simulink model "db3_6_Level_double"  (R2021a)
settings: Solver=VariableStepAuto  StartTime=0.0  StopTime=8  RelTol=1e-3
undefined symbols (not defined in the file): lambda2
libraries: dspsigops x13, dspquant2 x1
(part 1 of 3)
settings Model: Creator=Ruth Matienzo  LastModifiedBy=Ruth Matienzo

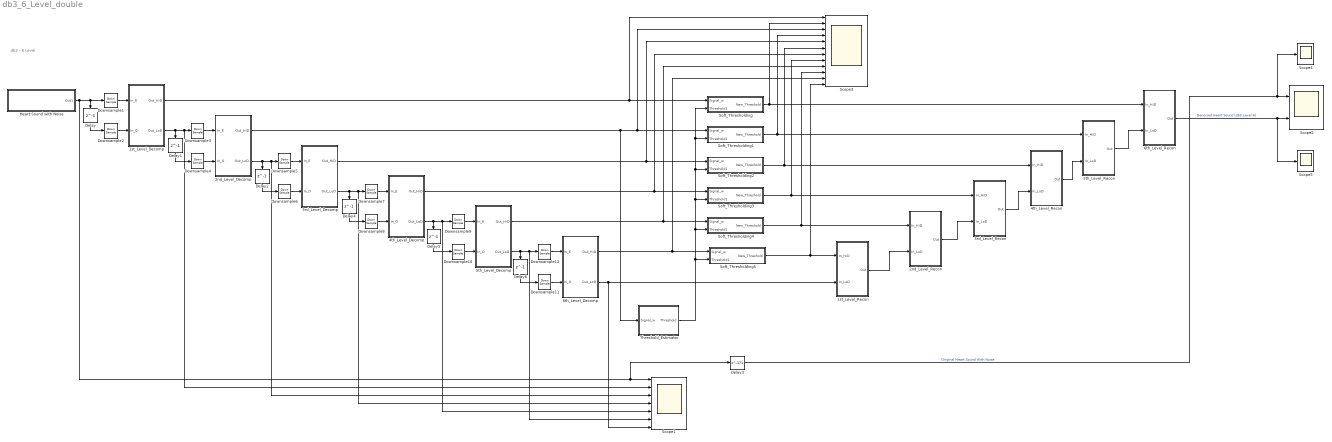
== system db3_6_Level_double ==
  note: db3 - 6 Level
  1st_Level_Decomp : Subsystem
  1st_Level_Recon : Subsystem
  2nd_Level_Decomp : Subsystem
  2nd_Level_Recon : Subsystem
  3rd_Level_Decomp : Subsystem
  3rd_Level_Recon : Subsystem
  4th_Level_Decomp : Subsystem
  4th_Level_Recon : Subsystem
  5th_Level_Decomp : Subsystem
  5th_Level_Recon : Subsystem
  6th_Level_Decomp : Subsystem
  6th_Level_Recon : Subsystem
  Delay{,1..2,4..6} (6 alike) : Delay  DelayLength=1  SampleTime=1/44100
  Delay3 : Delay  DelayLength=171  SampleTime=1/44100
  Downsample{1..12} (12 alike) : DownSample  N=30
  Heart Sound with Noise : Subsystem
  Scope1 : Scope  NumInputPorts=7
  Scope2 : Scope  NumInputPorts=2
  Scope3 : Scope  NumInputPorts=12
  Scope4 : Scope
  Scope5 : Scope
  Soft_Thresholding : Subsystem
  Soft_Thresholding1 : Subsystem
  Soft_Thresholding2 : Subsystem
  Soft_Thresholding3 : Subsystem
  Soft_Thresholding4 : Subsystem
  Soft_Thresholding5 : Subsystem
  Threshold_Estimator : Subsystem
  wires:
  1st_Level_Decomp/2(Out_LoD) -> Scope1/2, Downsample3/1, Delay1/1
  Downsample5/1 -> 3rd_Level_Decomp/1(In_E)
  Downsample8/1 -> 4th_Level_Decomp/2(In_O)
  Heart Sound with Noise/1(Out1) -> Downsample1/1, Delay/1, Delay3/1, Scope1/1
  Downsample3/1 -> 2nd_Level_Decomp/1(In_E)
  Delay2/1 -> Downsample6/1
  Downsample1/1 -> 1st_Level_Decomp/1(In_E)
  2nd_Level_Decomp/1(Out_HiD) -> Threshold_Estimator/1(Signal_w), Soft_Thresholding1/1(Signal_w), Scope3/3
  1st_Level_Decomp/1(Out_HiD) -> Soft_Thresholding/1(Signal_w), Scope3/1
  Soft_Thresholding1/1(New_Threshold) -> 5th_Level_Recon/1(In_HiD), Scope3/4
  Soft_Thresholding2/1(New_Threshold) -> 4th_Level_Recon/1(In_HiD), Scope3/6
  Downsample7/1 -> 4th_Level_Decomp/1(In_E)
  Soft_Thresholding/1(New_Threshold) -> 6th_Level_Recon/1(In_HiD), Scope3/2
  Downsample2/1 -> 1st_Level_Decomp/2(In_O)
  Downsample6/1 -> 3rd_Level_Decomp/2(In_O)
  Delay4/1 -> Downsample8/1
  Soft_Thresholding3/1(New_Threshold) -> 3rd_Level_Recon/1(In_HiD), Scope3/8
  Delay/1 -> Downsample2/1
  3rd_Level_Decomp/1(Out_HiD) -> Soft_Thresholding2/1(Signal_w), Scope3/5
  3rd_Level_Recon/1(Out) -> 4th_Level_Recon/2(In_LoD)
  4th_Level_Decomp/1(Out_HiD) -> Soft_Thresholding3/1(Signal_w), Scope3/7
  5th_Level_Recon/1(Out) -> 6th_Level_Recon/2(In_LoD)
  Downsample9/1 -> 5th_Level_Decomp/1(In_E)
  Delay5/1 -> Downsample10/1
  2nd_Level_Decomp/2(Out_LoD) -> Scope1/3, Downsample5/1, Delay2/1
  4th_Level_Recon/1(Out) -> 5th_Level_Recon/2(In_LoD)
  Threshold_Estimator/1(Threshold) -> Soft_Thresholding4/2(Threshold1), Soft_Thresholding1/2(Threshold1), Soft_Thresholding/2(Threshold1), Soft_Thresholding2/2(Threshold1), Soft_Thresholding3/2(Threshold1), Soft_Thresholding5/2(Threshold1)
  Delay1/1 -> Downsample4/1
  3rd_Level_Decomp/2(Out_LoD) -> Scope1/4, Downsample7/1, Delay4/1
  Downsample4/1 -> 2nd_Level_Decomp/2(In_O)
  Downsample10/1 -> 5th_Level_Decomp/2(In_O)
  4th_Level_Decomp/2(Out_LoD) -> Scope1/5, Downsample9/1, Delay5/1
  2nd_Level_Recon/1(Out) -> 3rd_Level_Recon/2(In_LoD)
  Soft_Thresholding4/1(New_Threshold) -> 2nd_Level_Recon/1(In_HiD), Scope3/10
  5th_Level_Decomp/1(Out_HiD) -> Scope3/9, Soft_Thresholding4/1(Signal_w)
  5th_Level_Decomp/2(Out_LoD) -> Scope1/6, Downsample12/1, Delay6/1
  Downsample11/1 -> 6th_Level_Decomp/2(In_O)
  Delay6/1 -> Downsample11/1
  Downsample12/1 -> 6th_Level_Decomp/1(In_E)
  6th_Level_Decomp/2(Out_LoD) -> 1st_Level_Recon/2(In_LoD), Scope1/7
  6th_Level_Decomp/1(Out_HiD) -> Scope3/11, Soft_Thresholding5/1(Signal_w)
  Soft_Thresholding5/1(New_Threshold) -> 1st_Level_Recon/1(In_HiD), Scope3/12
  1st_Level_Recon/1(Out) -> 2nd_Level_Recon/2(In_LoD)
  Delay3/1 -> Scope4/1, Scope2/1  "Original Heart Sound With Noise"
  6th_Level_Recon/1(Out) -> Scope5/1, Scope2/2  "Denoised Heart Sound (db3 Level 6)"

== system db3_6_Level_double/1st_Level_Decomp ==
  In_E : Inport  OutDataTypeStr=double  SampleTime=1/44100
  In_O : Inport  Port=2  OutDataTypeStr=double  SampleTime=1/44100
  Add : Sum  AccumDataTypeStr=double  OutDataTypeStr=double
  Add1 : Sum  AccumDataTypeStr=double  OutDataTypeStr=double
  Delay1 : Delay  DelayLength=1  SampleTime=1/44100
  Delay2 : Delay  DelayLength=1  SampleTime=1/44100
  Divide1 : Product  Inputs=*/  OutDataTypeStr=double
  Divide2 : Product  Inputs=*/  OutDataTypeStr=double
  HiD : Constant  Value=0.877989329+0.977128821  OutDataTypeStr=double  SampleTime=1/44100
  HiD_Even : Subsystem
  HiD_Odd : Subsystem
  LoD : Constant  Value=0.977128821+0.877989329  OutDataTypeStr=double  SampleTime=1/44100
  LoD_Even : Subsystem
  LoD_Odd : Subsystem
  Out_HiD : Outport  OutDataTypeStr=double  SampleTime=1/44100
  Out_LoD : Outport  Port=2  OutDataTypeStr=double  SampleTime=1/44100
  wires:
  HiD_Even/1(Out_HiD_e) -> Add/1
  HiD_Odd/1(Out_HiD_o) -> Add/2
  LoD_Odd/1(Out_LoD_o) -> Add1/2
  LoD_Even/1(Out_LoD_e) -> Add1/1
  In_E/1 -> HiD_Even/1(In_HiD_e), LoD_Even/1(In_LoD_e)
  In_O/1 -> LoD_Odd/1(In_LoD_o), HiD_Odd/1(In_HiD_o)
  HiD/1 -> Divide1/2
  Add1/1 -> Divide2/1
  LoD/1 -> Divide2/2
  Add/1 -> Divide1/1
  Delay1/1 -> Out_HiD/1
  Divide1/1 -> Delay1/1
  Delay2/1 -> Out_LoD/1
  Divide2/1 -> Delay2/1

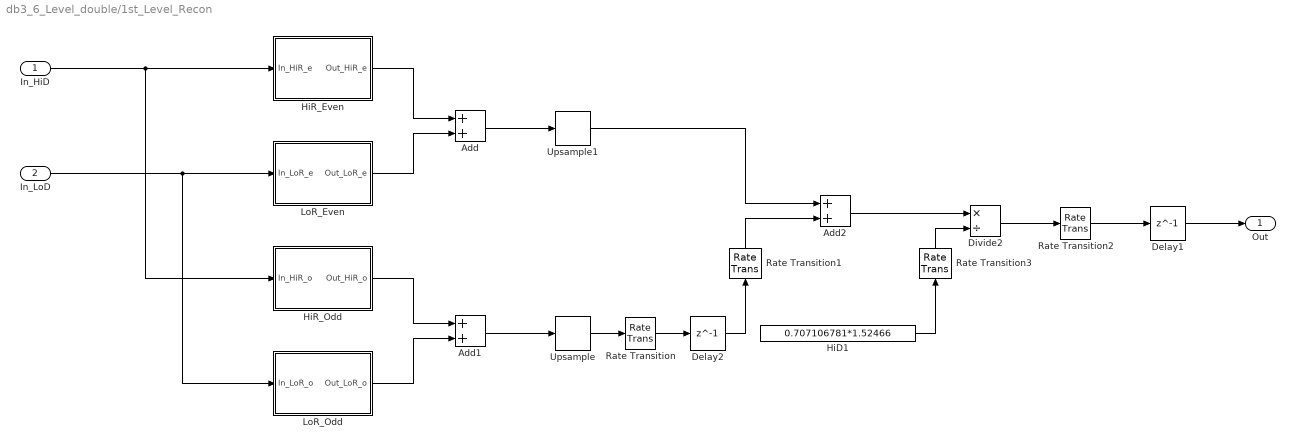
== system db3_6_Level_double/1st_Level_Recon ==
  In_HiD : Inport  OutDataTypeStr=double  SampleTime=1/44100
  In_LoD : Inport  Port=2  OutDataTypeStr=double  SampleTime=1/44100
  Add : Sum  AccumDataTypeStr=double  OutDataTypeStr=double
  Add1 : Sum  AccumDataTypeStr=double  OutDataTypeStr=double
  Add2 : Sum  AccumDataTypeStr=double  OutDataTypeStr=double
  Delay1 : Delay  DelayLength=1  SampleTime=1/44100
  Delay2 : Delay  DelayLength=1  SampleTime=1/44100
  Divide2 : Product  Inputs=*/  OutDataTypeStr=double  RndMeth=Zero  SaturateOnIntegerOverflow=on
  HiD1 : Constant  Value=0.707106781*1.52466  OutDataTypeStr=double  SampleTime=1/44100
  HiR_Even : Subsystem
  HiR_Odd : Subsystem
  LoR_Even : Subsystem
  LoR_Odd : Subsystem
  Rate Transition{,1..3} (4 alike) : RateTransition  OutPortSampleTime=1/44100
  Upsample : dspsigops/Upsample  N=30  phase=0  RateOptions=Allow multirate processing  ic=0  mode=Unused parameter value
  Upsample1 : dspsigops/Upsample  N=30  phase=0  RateOptions=Allow multirate processing  ic=0  mode=Unused parameter value
  Out : Outport  OutDataTypeStr=double  SampleTime=1/44100
  wires:
  In_HiD/1 -> HiR_Odd/1(In_HiR_o), HiR_Even/1(In_HiR_e)
  Add/1 -> Upsample1/1
  Add1/1 -> Upsample/1
  Upsample/1 -> Rate Transition/1
  Upsample1/1 -> Add2/1
  Delay2/1 -> Rate Transition1/1
  HiR_Even/1(Out_HiR_e) -> Add/1
  In_LoD/1 -> LoR_Odd/1(In_LoR_o), LoR_Even/1(In_LoR_e)
  LoR_Even/1(Out_LoR_e) -> Add/2
  HiR_Odd/1(Out_HiR_o) -> Add1/1
  LoR_Odd/1(Out_LoR_o) -> Add1/2
  Rate Transition/1 -> Delay2/1
  Rate Transition1/1 -> Add2/2
  Rate Transition2/1 -> Delay1/1
  Delay1/1 -> Out/1
  HiD1/1 -> Rate Transition3/1
  Add2/1 -> Divide2/1
  Divide2/1 -> Rate Transition2/1
  Rate Transition3/1 -> Divide2/2

== system db3_6_Level_double/2nd_Level_Decomp ==
  In_E : Inport  OutDataTypeStr=double  SampleTime=1/44100
  In_O : Inport  Port=2  OutDataTypeStr=double  SampleTime=1/44100
  Add : Sum  AccumDataTypeStr=double  OutDataTypeStr=double
  Add1 : Sum  AccumDataTypeStr=double  OutDataTypeStr=double
  Delay1 : Delay  DelayLength=1  SampleTime=1/44100
  Delay2 : Delay  DelayLength=1  SampleTime=1/44100
  Divide1 : Product  Inputs=*/  OutDataTypeStr=double
  Divide2 : Product  Inputs=*/  OutDataTypeStr=double
  HiD : Constant  Value=0.877989329+0.977128821  OutDataTypeStr=double  SampleTime=1/44100
  HiD_Even : Subsystem
  HiD_Odd : Subsystem
  LoD : Constant  Value=0.977128821+0.877989329  OutDataTypeStr=double  SampleTime=1/44100
  LoD_Even : Subsystem
  LoD_Odd : Subsystem
  Out_HiD : Outport  OutDataTypeStr=double  SampleTime=1/44100
  Out_LoD : Outport  Port=2  OutDataTypeStr=double  SampleTime=1/44100
  wires:
  HiD_Even/1(Out_HiD_e) -> Add/1
  HiD_Odd/1(Out_HiD_o) -> Add/2
  LoD_Odd/1(Out_LoD_o) -> Add1/2
  LoD_Even/1(Out_LoD_e) -> Add1/1
  In_E/1 -> HiD_Even/1(In_HiD_e), LoD_Even/1(In_LoD_e)
  In_O/1 -> LoD_Odd/1(In_LoD_o), HiD_Odd/1(In_HiD_o)
  HiD/1 -> Divide1/2
  Add1/1 -> Divide2/1
  LoD/1 -> Divide2/2
  Add/1 -> Divide1/1
  Delay1/1 -> Out_HiD/1
  Divide1/1 -> Delay1/1
  Delay2/1 -> Out_LoD/1
  Divide2/1 -> Delay2/1

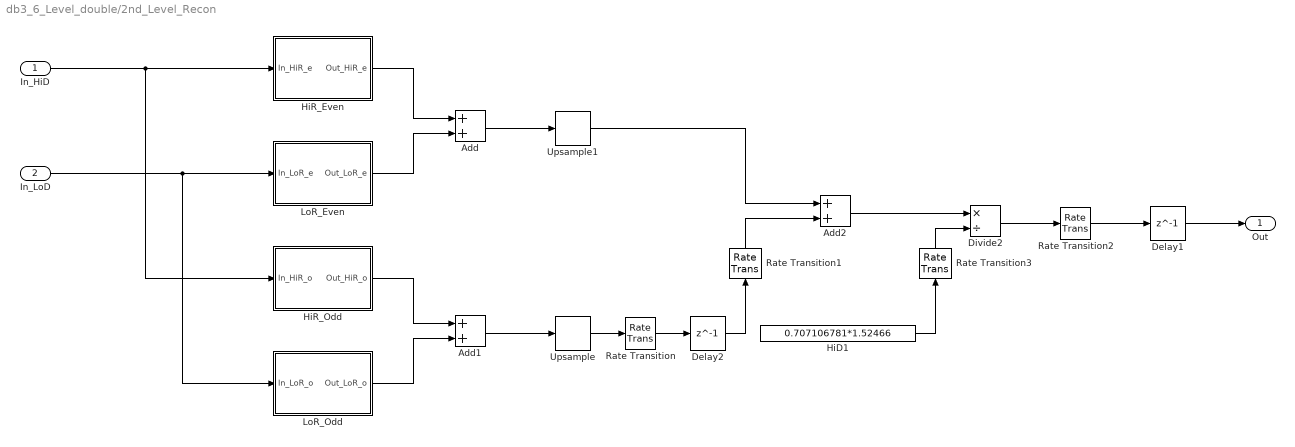
== system db3_6_Level_double/2nd_Level_Recon ==
  In_HiD : Inport  OutDataTypeStr=double  SampleTime=1/44100
  In_LoD : Inport  Port=2  OutDataTypeStr=double  SampleTime=1/44100
  Add : Sum  AccumDataTypeStr=double  OutDataTypeStr=double
  Add1 : Sum  AccumDataTypeStr=double  OutDataTypeStr=double
  Add2 : Sum  AccumDataTypeStr=double  OutDataTypeStr=double
  Delay1 : Delay  DelayLength=1  SampleTime=1/44100
  Delay2 : Delay  DelayLength=1  SampleTime=1/44100
  Divide2 : Product  Inputs=*/  OutDataTypeStr=double  RndMeth=Zero  SaturateOnIntegerOverflow=on
  HiD1 : Constant  Value=0.707106781*1.52466  OutDataTypeStr=double  SampleTime=1/44100
  HiR_Even : Subsystem
  HiR_Odd : Subsystem
  LoR_Even : Subsystem
  LoR_Odd : Subsystem
  Rate Transition{,1..3} (4 alike) : RateTransition  OutPortSampleTime=1/44100
  Upsample : dspsigops/Upsample  N=30  phase=0  RateOptions=Allow multirate processing  ic=0  mode=Unused parameter value
  Upsample1 : dspsigops/Upsample  N=30  phase=0  RateOptions=Allow multirate processing  ic=0  mode=Unused parameter value
  Out : Outport  OutDataTypeStr=double  SampleTime=1/44100
  wires:
  In_HiD/1 -> HiR_Odd/1(In_HiR_o), HiR_Even/1(In_HiR_e)
  Add/1 -> Upsample1/1
  Add1/1 -> Upsample/1
  Upsample/1 -> Rate Transition/1
  Upsample1/1 -> Add2/1
  Delay2/1 -> Rate Transition1/1
  HiR_Even/1(Out_HiR_e) -> Add/1
  In_LoD/1 -> LoR_Odd/1(In_LoR_o), LoR_Even/1(In_LoR_e)
  LoR_Even/1(Out_LoR_e) -> Add/2
  HiR_Odd/1(Out_HiR_o) -> Add1/1
  LoR_Odd/1(Out_LoR_o) -> Add1/2
  Rate Transition/1 -> Delay2/1
  Rate Transition1/1 -> Add2/2
  Rate Transition2/1 -> Delay1/1
  Delay1/1 -> Out/1
  HiD1/1 -> Rate Transition3/1
  Add2/1 -> Divide2/1
  Divide2/1 -> Rate Transition2/1
  Rate Transition3/1 -> Divide2/2

== system db3_6_Level_double/3rd_Level_Decomp ==
  In_E : Inport  OutDataTypeStr=double  SampleTime=1/44100
  In_O : Inport  Port=2  OutDataTypeStr=double  SampleTime=1/44100
  Add : Sum  AccumDataTypeStr=double  OutDataTypeStr=double
  Add1 : Sum  AccumDataTypeStr=double  OutDataTypeStr=double
  Delay1 : Delay  DelayLength=1  SampleTime=1/44100
  Delay2 : Delay  DelayLength=1  SampleTime=1/44100
  Divide1 : Product  Inputs=*/  OutDataTypeStr=double
  Divide2 : Product  Inputs=*/  OutDataTypeStr=double
  HiD : Constant  Value=0.877989329+0.977128821  OutDataTypeStr=double  SampleTime=1/44100
  HiD_Even : Subsystem
  HiD_Odd : Subsystem
  LoD : Constant  Value=0.977128821+0.877989329  OutDataTypeStr=double  SampleTime=1/44100
  LoD_Even : Subsystem
  LoD_Odd : Subsystem
  Out_HiD : Outport  OutDataTypeStr=double  SampleTime=1/44100
  Out_LoD : Outport  Port=2  OutDataTypeStr=double  SampleTime=1/44100
  wires:
  HiD_Even/1(Out_HiD_e) -> Add/1
  HiD_Odd/1(Out_HiD_o) -> Add/2
  LoD_Odd/1(Out_LoD_o) -> Add1/2
  LoD_Even/1(Out_LoD_e) -> Add1/1
  In_E/1 -> HiD_Even/1(In_HiD_e), LoD_Even/1(In_LoD_e)
  In_O/1 -> LoD_Odd/1(In_LoD_o), HiD_Odd/1(In_HiD_o)
  HiD/1 -> Divide1/2
  Add1/1 -> Divide2/1
  LoD/1 -> Divide2/2
  Add/1 -> Divide1/1
  Delay1/1 -> Out_HiD/1
  Divide1/1 -> Delay1/1
  Delay2/1 -> Out_LoD/1
  Divide2/1 -> Delay2/1

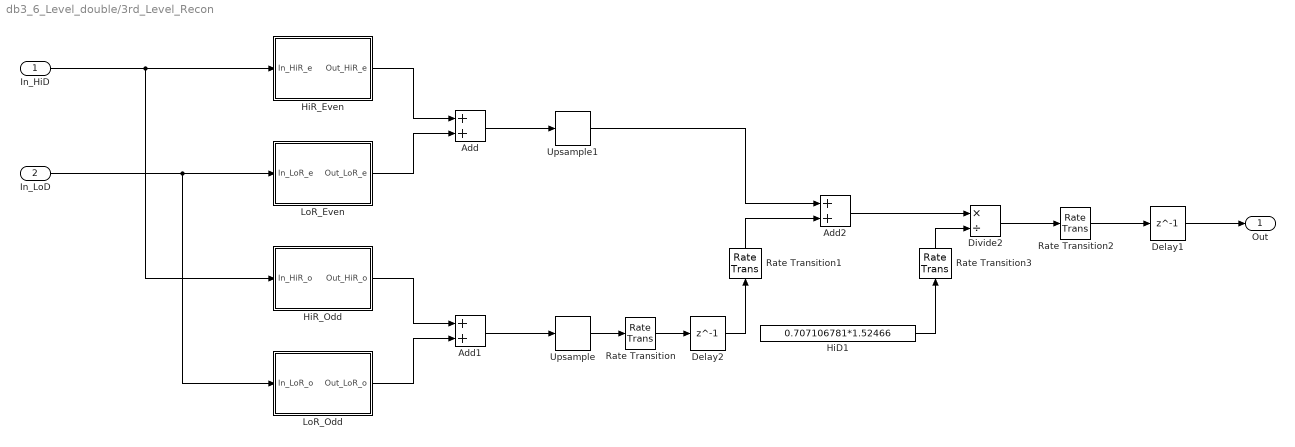
== system db3_6_Level_double/3rd_Level_Recon ==
  In_HiD : Inport  OutDataTypeStr=double  SampleTime=1/44100
  In_LoD : Inport  Port=2  OutDataTypeStr=double  SampleTime=1/44100
  Add : Sum  AccumDataTypeStr=double  OutDataTypeStr=double
  Add1 : Sum  AccumDataTypeStr=double  OutDataTypeStr=double
  Add2 : Sum  AccumDataTypeStr=double  OutDataTypeStr=double
  Delay1 : Delay  DelayLength=1  SampleTime=1/44100
  Delay2 : Delay  DelayLength=1  SampleTime=1/44100
  Divide2 : Product  Inputs=*/  OutDataTypeStr=double  RndMeth=Zero  SaturateOnIntegerOverflow=on
  HiD1 : Constant  Value=0.707106781*1.52466  OutDataTypeStr=double  SampleTime=1/44100
  HiR_Even : Subsystem
  HiR_Odd : Subsystem
  LoR_Even : Subsystem
  LoR_Odd : Subsystem
  Rate Transition{,1..3} (4 alike) : RateTransition  OutPortSampleTime=1/44100
  Upsample : dspsigops/Upsample  N=30  phase=0  RateOptions=Allow multirate processing  ic=0  mode=Unused parameter value
  Upsample1 : dspsigops/Upsample  N=30  phase=0  RateOptions=Allow multirate processing  ic=0  mode=Unused parameter value
  Out : Outport  OutDataTypeStr=double  SampleTime=1/44100
  wires:
  In_HiD/1 -> HiR_Odd/1(In_HiR_o), HiR_Even/1(In_HiR_e)
  Add/1 -> Upsample1/1
  Add1/1 -> Upsample/1
  Upsample/1 -> Rate Transition/1
  Upsample1/1 -> Add2/1
  Delay2/1 -> Rate Transition1/1
  HiR_Even/1(Out_HiR_e) -> Add/1
  In_LoD/1 -> LoR_Odd/1(In_LoR_o), LoR_Even/1(In_LoR_e)
  LoR_Even/1(Out_LoR_e) -> Add/2
  HiR_Odd/1(Out_HiR_o) -> Add1/1
  LoR_Odd/1(Out_LoR_o) -> Add1/2
  Rate Transition/1 -> Delay2/1
  Rate Transition1/1 -> Add2/2
  Rate Transition2/1 -> Delay1/1
  Delay1/1 -> Out/1
  HiD1/1 -> Rate Transition3/1
  Add2/1 -> Divide2/1
  Divide2/1 -> Rate Transition2/1
  Rate Transition3/1 -> Divide2/2

== system db3_6_Level_double/4th_Level_Decomp ==
  In_E : Inport  OutDataTypeStr=double  SampleTime=1/44100
  In_O : Inport  Port=2  OutDataTypeStr=double  SampleTime=1/44100
  Add : Sum  AccumDataTypeStr=double  OutDataTypeStr=double
  Add1 : Sum  AccumDataTypeStr=double  OutDataTypeStr=double
  Delay1 : Delay  DelayLength=1  SampleTime=1/44100
  Delay2 : Delay  DelayLength=1  SampleTime=1/44100
  Divide1 : Product  Inputs=*/  OutDataTypeStr=double
  Divide2 : Product  Inputs=*/  OutDataTypeStr=double
  HiD : Constant  Value=0.877989329+0.977128821  OutDataTypeStr=double  SampleTime=1/44100
  HiD_Even : Subsystem
  HiD_Odd : Subsystem
  LoD : Constant  Value=0.977128821+0.877989329  OutDataTypeStr=double  SampleTime=1/44100
  LoD_Even : Subsystem
  LoD_Odd : Subsystem
  Out_HiD : Outport  OutDataTypeStr=double  SampleTime=1/44100
  Out_LoD : Outport  Port=2  OutDataTypeStr=double  SampleTime=1/44100
  wires:
  HiD_Even/1(Out_HiD_e) -> Add/1
  HiD_Odd/1(Out_HiD_o) -> Add/2
  LoD_Odd/1(Out_LoD_o) -> Add1/2
  LoD_Even/1(Out_LoD_e) -> Add1/1
  In_E/1 -> HiD_Even/1(In_HiD_e), LoD_Even/1(In_LoD_e)
  In_O/1 -> LoD_Odd/1(In_LoD_o), HiD_Odd/1(In_HiD_o)
  HiD/1 -> Divide1/2
  Add1/1 -> Divide2/1
  LoD/1 -> Divide2/2
  Add/1 -> Divide1/1
  Delay1/1 -> Out_HiD/1
  Divide1/1 -> Delay1/1
  Delay2/1 -> Out_LoD/1
  Divide2/1 -> Delay2/1

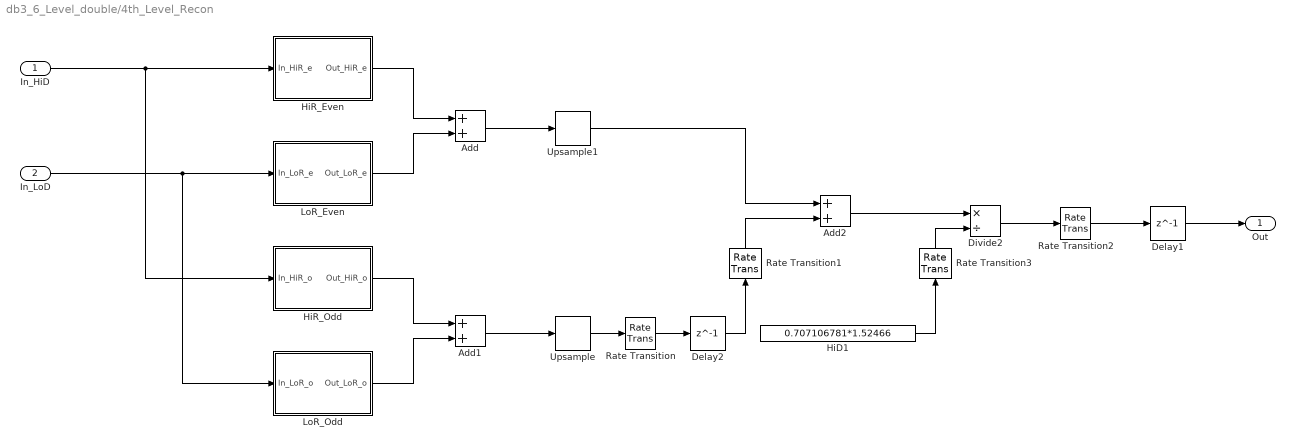
== system db3_6_Level_double/4th_Level_Recon ==
  In_HiD : Inport  OutDataTypeStr=double  SampleTime=1/44100
  In_LoD : Inport  Port=2  OutDataTypeStr=double  SampleTime=1/44100
  Add : Sum  AccumDataTypeStr=double  OutDataTypeStr=double
  Add1 : Sum  AccumDataTypeStr=double  OutDataTypeStr=double
  Add2 : Sum  AccumDataTypeStr=double  OutDataTypeStr=double
  Delay1 : Delay  DelayLength=1  SampleTime=1/44100
  Delay2 : Delay  DelayLength=1  SampleTime=1/44100
  Divide2 : Product  Inputs=*/  OutDataTypeStr=double  RndMeth=Zero  SaturateOnIntegerOverflow=on
  HiD1 : Constant  Value=0.707106781*1.52466  OutDataTypeStr=double  SampleTime=1/44100
  HiR_Even : Subsystem
  HiR_Odd : Subsystem
  LoR_Even : Subsystem
  LoR_Odd : Subsystem
  Rate Transition{,1..3} (4 alike) : RateTransition  OutPortSampleTime=1/44100
  Upsample : dspsigops/Upsample  N=30  phase=0  RateOptions=Allow multirate processing  ic=0  mode=Unused parameter value
  Upsample1 : dspsigops/Upsample  N=30  phase=0  RateOptions=Allow multirate processing  ic=0  mode=Unused parameter value
  Out : Outport  OutDataTypeStr=double  SampleTime=1/44100
  wires:
  In_HiD/1 -> HiR_Odd/1(In_HiR_o), HiR_Even/1(In_HiR_e)
  Add/1 -> Upsample1/1
  Add1/1 -> Upsample/1
  Upsample/1 -> Rate Transition/1
  Upsample1/1 -> Add2/1
  Delay2/1 -> Rate Transition1/1
  HiR_Even/1(Out_HiR_e) -> Add/1
  In_LoD/1 -> LoR_Odd/1(In_LoR_o), LoR_Even/1(In_LoR_e)
  LoR_Even/1(Out_LoR_e) -> Add/2
  HiR_Odd/1(Out_HiR_o) -> Add1/1
  LoR_Odd/1(Out_LoR_o) -> Add1/2
  Rate Transition/1 -> Delay2/1
  Rate Transition1/1 -> Add2/2
  Rate Transition2/1 -> Delay1/1
  Delay1/1 -> Out/1
  HiD1/1 -> Rate Transition3/1
  Add2/1 -> Divide2/1
  Divide2/1 -> Rate Transition2/1
  Rate Transition3/1 -> Divide2/2

== system db3_6_Level_double/5th_Level_Decomp ==
  In_E : Inport  OutDataTypeStr=double  SampleTime=1/44100
  In_O : Inport  Port=2  OutDataTypeStr=double  SampleTime=1/44100
  Add : Sum  AccumDataTypeStr=double  OutDataTypeStr=double
  Add1 : Sum  AccumDataTypeStr=double  OutDataTypeStr=double
  Delay1 : Delay  DelayLength=1  SampleTime=1/44100
  Delay2 : Delay  DelayLength=1  SampleTime=1/44100
  Divide1 : Product  Inputs=*/  OutDataTypeStr=double
  Divide2 : Product  Inputs=*/  OutDataTypeStr=double
  HiD : Constant  Value=0.877989329+0.977128821  OutDataTypeStr=double  SampleTime=1/44100
  HiD_Even : Subsystem
  HiD_Odd : Subsystem
  LoD : Constant  Value=0.977128821+0.877989329  OutDataTypeStr=double  SampleTime=1/44100
  LoD_Even : Subsystem
  LoD_Odd : Subsystem
  Out_HiD : Outport  OutDataTypeStr=double  SampleTime=1/44100
  Out_LoD : Outport  Port=2  OutDataTypeStr=double  SampleTime=1/44100
  wires:
  HiD_Even/1(Out_HiD_e) -> Add/1
  HiD_Odd/1(Out_HiD_o) -> Add/2
  LoD_Odd/1(Out_LoD_o) -> Add1/2
  LoD_Even/1(Out_LoD_e) -> Add1/1
  In_E/1 -> HiD_Even/1(In_HiD_e), LoD_Even/1(In_LoD_e)
  In_O/1 -> LoD_Odd/1(In_LoD_o), HiD_Odd/1(In_HiD_o)
  HiD/1 -> Divide1/2
  Add1/1 -> Divide2/1
  LoD/1 -> Divide2/2
  Add/1 -> Divide1/1
  Delay1/1 -> Out_HiD/1
  Divide1/1 -> Delay1/1
  Delay2/1 -> Out_LoD/1
  Divide2/1 -> Delay2/1

== system db3_6_Level_double/5th_Level_Recon ==
  In_HiD : Inport  OutDataTypeStr=double  SampleTime=1/44100
  In_LoD : Inport  Port=2  OutDataTypeStr=double  SampleTime=1/44100
  Add : Sum  AccumDataTypeStr=double  OutDataTypeStr=double
  Add1 : Sum  AccumDataTypeStr=double  OutDataTypeStr=double
  Add2 : Sum  AccumDataTypeStr=double  OutDataTypeStr=double
  Delay1 : Delay  DelayLength=1  SampleTime=1/44100
  Delay2 : Delay  DelayLength=1  SampleTime=1/44100
  Divide2 : Product  Inputs=*/  OutDataTypeStr=double  RndMeth=Zero  SaturateOnIntegerOverflow=on
  HiD1 : Constant  Value=0.707106781*1.52466  OutDataTypeStr=double  SampleTime=1/44100
  HiR_Even : Subsystem
  HiR_Odd : Subsystem
  LoR_Even : Subsystem
  LoR_Odd : Subsystem
  Rate Transition{,1..3} (4 alike) : RateTransition  OutPortSampleTime=1/44100
  Upsample : dspsigops/Upsample  N=30  phase=0  RateOptions=Allow multirate processing  ic=0  mode=Unused parameter value
  Upsample1 : dspsigops/Upsample  N=30  phase=0  RateOptions=Allow multirate processing  ic=0  mode=Unused parameter value
  Out : Outport  OutDataTypeStr=double  SampleTime=1/44100
  wires:
  In_HiD/1 -> HiR_Odd/1(In_HiR_o), HiR_Even/1(In_HiR_e)
  Add/1 -> Upsample1/1
  Add1/1 -> Upsample/1
  Upsample/1 -> Rate Transition/1
  Upsample1/1 -> Add2/1
  Delay2/1 -> Rate Transition1/1
  HiR_Even/1(Out_HiR_e) -> Add/1
  In_LoD/1 -> LoR_Odd/1(In_LoR_o), LoR_Even/1(In_LoR_e)
  LoR_Even/1(Out_LoR_e) -> Add/2
  HiR_Odd/1(Out_HiR_o) -> Add1/1
  LoR_Odd/1(Out_LoR_o) -> Add1/2
  Rate Transition/1 -> Delay2/1
  Rate Transition1/1 -> Add2/2
  Rate Transition2/1 -> Delay1/1
  Delay1/1 -> Out/1
  HiD1/1 -> Rate Transition3/1
  Add2/1 -> Divide2/1
  Divide2/1 -> Rate Transition2/1
  Rate Transition3/1 -> Divide2/2

== system db3_6_Level_double/6th_Level_Decomp ==
  In_E : Inport  OutDataTypeStr=double  SampleTime=1/44100
  In_O : Inport  Port=2  OutDataTypeStr=double  SampleTime=1/44100
  Add : Sum  AccumDataTypeStr=double  OutDataTypeStr=double
  Add1 : Sum  AccumDataTypeStr=double  OutDataTypeStr=double
  Delay1 : Delay  DelayLength=1  SampleTime=1/44100
  Delay2 : Delay  DelayLength=1  SampleTime=1/44100
  Divide1 : Product  Inputs=*/  OutDataTypeStr=double
  Divide2 : Product  Inputs=*/  OutDataTypeStr=double
  HiD : Constant  Value=0.877989329+0.977128821  OutDataTypeStr=double  SampleTime=1/44100
  HiD_Even : Subsystem
  HiD_Odd : Subsystem
  LoD : Constant  Value=0.977128821+0.877989329  OutDataTypeStr=double  SampleTime=1/44100
  LoD_Even : Subsystem
  LoD_Odd : Subsystem
  Out_HiD : Outport  OutDataTypeStr=double  SampleTime=1/44100
  Out_LoD : Outport  Port=2  OutDataTypeStr=double  SampleTime=1/44100
  wires:
  HiD_Even/1(Out_HiD_e) -> Add/1
  HiD_Odd/1(Out_HiD_o) -> Add/2
  LoD_Odd/1(Out_LoD_o) -> Add1/2
  LoD_Even/1(Out_LoD_e) -> Add1/1
  In_E/1 -> HiD_Even/1(In_HiD_e), LoD_Even/1(In_LoD_e)
  In_O/1 -> LoD_Odd/1(In_LoD_o), HiD_Odd/1(In_HiD_o)
  HiD/1 -> Divide1/2
  Add1/1 -> Divide2/1
  LoD/1 -> Divide2/2
  Add/1 -> Divide1/1
  Delay1/1 -> Out_HiD/1
  Divide1/1 -> Delay1/1
  Delay2/1 -> Out_LoD/1
  Divide2/1 -> Delay2/1

== system db3_6_Level_double/6th_Level_Recon ==
  In_HiD : Inport  OutDataTypeStr=double  SampleTime=1/44100
  In_LoD : Inport  Port=2  OutDataTypeStr=double  SampleTime=1/44100
  Add : Sum  AccumDataTypeStr=double  OutDataTypeStr=double
  Add1 : Sum  AccumDataTypeStr=double  OutDataTypeStr=double
  Add2 : Sum  AccumDataTypeStr=double  OutDataTypeStr=double
  Delay1 : Delay  DelayLength=1  SampleTime=1/44100
  Delay2 : Delay  DelayLength=1  SampleTime=1/44100
  Divide2 : Product  Inputs=*/  OutDataTypeStr=double  RndMeth=Zero  SaturateOnIntegerOverflow=on
  HiD1 : Constant  Value=0.707106781*1.52466  OutDataTypeStr=double  SampleTime=1/44100
  HiR_Even : Subsystem
  HiR_Odd : Subsystem
  LoR_Even : Subsystem
  LoR_Odd : Subsystem
  Rate Transition{,1..3} (4 alike) : RateTransition  OutPortSampleTime=1/44100
  Upsample : dspsigops/Upsample  N=30  phase=0  RateOptions=Allow multirate processing  ic=0  mode=Unused parameter value
  Upsample1 : dspsigops/Upsample  N=30  phase=0  RateOptions=Allow multirate processing  ic=0  mode=Unused parameter value
  Out : Outport  OutDataTypeStr=double  SampleTime=1/44100
  wires:
  In_HiD/1 -> HiR_Odd/1(In_HiR_o), HiR_Even/1(In_HiR_e)
  Add/1 -> Upsample1/1
  Add1/1 -> Upsample/1
  Upsample/1 -> Rate Transition/1
  Upsample1/1 -> Add2/1
  Delay2/1 -> Rate Transition1/1
  HiR_Even/1(Out_HiR_e) -> Add/1
  In_LoD/1 -> LoR_Odd/1(In_LoR_o), LoR_Even/1(In_LoR_e)
  LoR_Even/1(Out_LoR_e) -> Add/2
  HiR_Odd/1(Out_HiR_o) -> Add1/1
  LoR_Odd/1(Out_LoR_o) -> Add1/2
  Rate Transition/1 -> Delay2/1
  Rate Transition1/1 -> Add2/2
  Rate Transition2/1 -> Delay1/1
  Delay1/1 -> Out/1
  HiD1/1 -> Rate Transition3/1
  Add2/1 -> Divide2/1
  Divide2/1 -> Rate Transition2/1
  Rate Transition3/1 -> Divide2/2

== system db3_6_Level_double/Heart Sound with Noise ==
  Constant : Constant  Value=80000  OutDataTypeStr=double  SampleTime=1/44100
  Divide : Product  Inputs=*/  OutDataTypeStr=double
  From Workspace1 : FromWorkspace  VariableName=Audio_Heart_Noise  OutDataTypeStr=double  SampleTime=1/44100
  Gain2 : Gain  Gain=5  ParamDataTypeStr=double  OutDataTypeStr=double
  Pulse Generator : DiscretePulseGenerator  PulseType=Time based  Period=0.00022675736  PulseWidth=50
  Quantizer : Quantizer  QuantizationInterval=0.1
  Sample and Hold : dspsigops/Sample and Hold  trig=Rising edge  initCond=0  latchinput=off
  Uniform Encoder : dspquant2/Uniform Encoder  peak=2  bits=8  otype=Unsigned integer
  Out1 : Outport  OutDataTypeStr=double  SampleTime=1/44100
  wires:
  Sample and Hold/1 -> Quantizer/1
  Uniform Encoder/1 -> Divide/1
  Quantizer/1 -> Uniform Encoder/1
  Constant/1 -> Divide/2
  From Workspace1/1 -> Gain2/1
  Pulse Generator/1 -> Sample and Hold/Trigger
  Gain2/1 -> Sample and Hold/1
  Divide/1 -> Out1/1

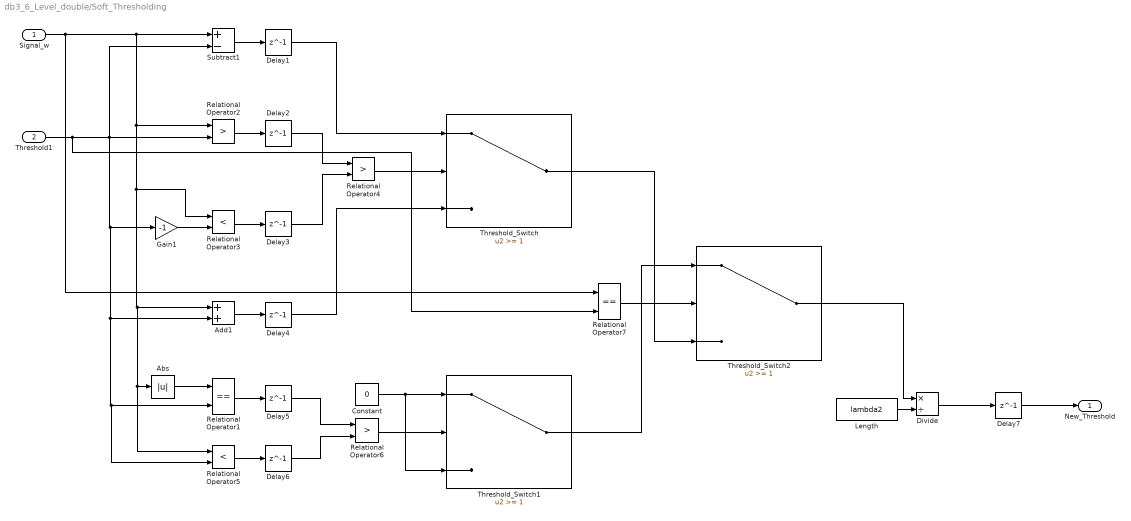
== system db3_6_Level_double/Soft_Thresholding ==
  Signal_w : Inport  OutDataTypeStr=double  SampleTime=1/44100
  Threshold1 : Inport  Port=2  OutDataTypeStr=double  SampleTime=1/44100
  Abs : Abs  OutDataTypeStr=double
  Add1 : Sum  AccumDataTypeStr=double  OutDataTypeStr=double
  Constant : Constant  Value=0  OutDataTypeStr=double  SampleTime=1/44100
  Delay{1..7} (7 alike) : Delay  DelayLength=1  SampleTime=1/44100
  Divide : Product  Inputs=*/  OutDataTypeStr=double
  Gain1 : Gain  Gain=-1  ParamDataTypeStr=double  OutMin=-1  OutMax=-0.99  OutDataTypeStr=double
  Length : Constant  Value=lambda2  OutDataTypeStr=double  SampleTime=1/44100
  Relational Operator1 : RelationalOperator  Operator===  OutDataTypeStr=boolean  RndMeth=Simplest
  Relational Operator2 : RelationalOperator  Operator=>  OutDataTypeStr=boolean  RndMeth=Simplest
  Relational Operator3 : RelationalOperator  Operator=<  OutDataTypeStr=boolean  RndMeth=Simplest
  Relational Operator4 : RelationalOperator  Operator=>  OutDataTypeStr=boolean  RndMeth=Simplest
  Relational Operator5 : RelationalOperator  Operator=<  OutDataTypeStr=boolean  RndMeth=Simplest
  Relational Operator6 : RelationalOperator  Operator=>  OutDataTypeStr=boolean  RndMeth=Simplest
  Relational Operator7 : RelationalOperator  Operator===  OutDataTypeStr=boolean  RndMeth=Simplest
  Subtract1 : Sum  Inputs=+-  AccumDataTypeStr=double  OutDataTypeStr=double
  Threshold_Switch : Switch  Threshold=1  OutDataTypeStr=double
  Threshold_Switch1 : Switch  Threshold=1  OutDataTypeStr=double
  Threshold_Switch2 : Switch  Threshold=1  OutDataTypeStr=double
  New_Threshold : Outport  OutDataTypeStr=double  SampleTime=1/44100
  wires:
  Threshold_Switch/1 -> Threshold_Switch2/3
  Relational Operator6/1 -> Threshold_Switch1/2
  Gain1/1 -> Relational Operator3/2
  Delay4/1 -> Threshold_Switch/3
  Add1/1 -> Delay4/1
  Delay2/1 -> Relational Operator4/1
  Delay3/1 -> Relational Operator4/2
  Delay1/1 -> Threshold_Switch/1
  Relational Operator2/1 -> Delay2/1
  Relational Operator3/1 -> Delay3/1
  Relational Operator5/1 -> Delay6/1
  Delay6/1 -> Relational Operator6/2
  Delay5/1 -> Relational Operator6/1
  Threshold1/1 -> Relational Operator2/2, Subtract1/2, Relational Operator5/2, Relational Operator1/2, Add1/2, Gain1/1, Relational Operator7/2
  Abs/1 -> Relational Operator1/1
  Relational Operator4/1 -> Threshold_Switch/2
  Subtract1/1 -> Delay1/1
  Constant/1 -> Threshold_Switch1/3, Threshold_Switch1/1
  Signal_w/1 -> Subtract1/1, Relational Operator2/1, Relational Operator5/1, Abs/1, Add1/1, Relational Operator3/1, Relational Operator7/1
  Relational Operator7/1 -> Threshold_Switch2/2
  Relational Operator1/1 -> Delay5/1
  Threshold_Switch1/1 -> Threshold_Switch2/1
  Threshold_Switch2/1 -> Divide/1
  Length/1 -> Divide/2
  Divide/1 -> Delay7/1
  Delay7/1 -> New_Threshold/1

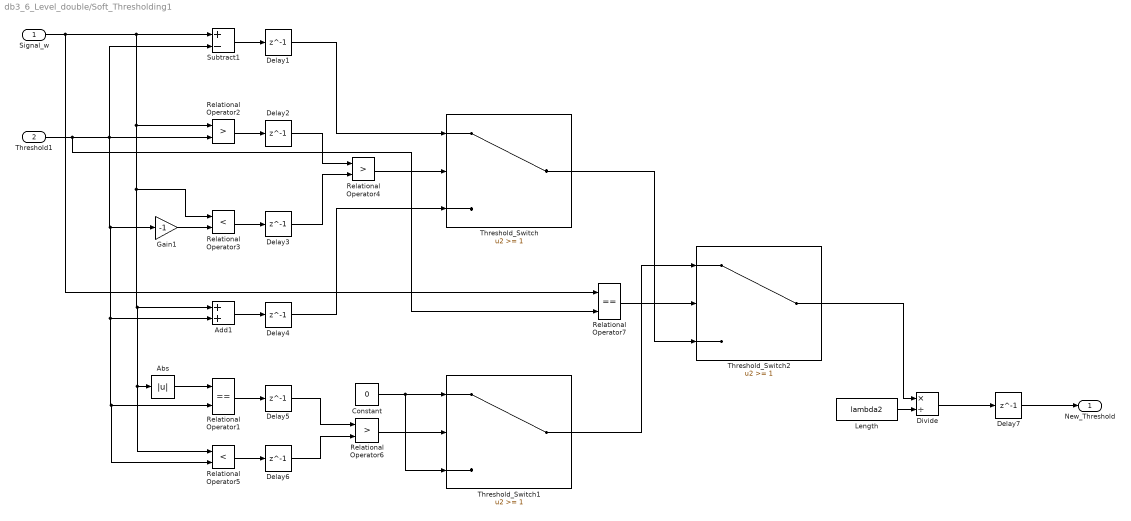
== system db3_6_Level_double/Soft_Thresholding1 ==
  Signal_w : Inport  OutDataTypeStr=double  SampleTime=1/44100
  Threshold1 : Inport  Port=2  OutDataTypeStr=double  SampleTime=1/44100
  Abs : Abs  OutDataTypeStr=double
  Add1 : Sum  AccumDataTypeStr=double  OutDataTypeStr=double
  Constant : Constant  Value=0  OutDataTypeStr=double  SampleTime=1/44100
  Delay{1..7} (7 alike) : Delay  DelayLength=1  SampleTime=1/44100
  Divide : Product  Inputs=*/  OutDataTypeStr=double
  Gain1 : Gain  Gain=-1  ParamDataTypeStr=double  OutMin=-1  OutMax=-0.99  OutDataTypeStr=double
  Length : Constant  Value=lambda2  OutDataTypeStr=double  SampleTime=1/44100
  Relational Operator1 : RelationalOperator  Operator===  OutDataTypeStr=boolean  RndMeth=Simplest
  Relational Operator2 : RelationalOperator  Operator=>  OutDataTypeStr=boolean  RndMeth=Simplest
  Relational Operator3 : RelationalOperator  Operator=<  OutDataTypeStr=boolean  RndMeth=Simplest
  Relational Operator4 : RelationalOperator  Operator=>  OutDataTypeStr=boolean  RndMeth=Simplest
  Relational Operator5 : RelationalOperator  Operator=<  OutDataTypeStr=boolean  RndMeth=Simplest
  Relational Operator6 : RelationalOperator  Operator=>  OutDataTypeStr=boolean  RndMeth=Simplest
  Relational Operator7 : RelationalOperator  Operator===  OutDataTypeStr=boolean  RndMeth=Simplest
  Subtract1 : Sum  Inputs=+-  AccumDataTypeStr=double  OutDataTypeStr=double
  Threshold_Switch : Switch  Threshold=1  OutDataTypeStr=double
  Threshold_Switch1 : Switch  Threshold=1  OutDataTypeStr=double
  Threshold_Switch2 : Switch  Threshold=1  OutDataTypeStr=double
  New_Threshold : Outport  OutDataTypeStr=double  SampleTime=1/44100
  wires:
  Threshold_Switch/1 -> Threshold_Switch2/3
  Relational Operator6/1 -> Threshold_Switch1/2
  Gain1/1 -> Relational Operator3/2
  Delay4/1 -> Threshold_Switch/3
  Add1/1 -> Delay4/1
  Delay2/1 -> Relational Operator4/1
  Delay3/1 -> Relational Operator4/2
  Delay1/1 -> Threshold_Switch/1
  Relational Operator2/1 -> Delay2/1
  Relational Operator3/1 -> Delay3/1
  Relational Operator5/1 -> Delay6/1
  Delay6/1 -> Relational Operator6/2
  Delay5/1 -> Relational Operator6/1
  Threshold1/1 -> Relational Operator2/2, Subtract1/2, Relational Operator5/2, Relational Operator1/2, Add1/2, Gain1/1, Relational Operator7/2
  Abs/1 -> Relational Operator1/1
  Relational Operator4/1 -> Threshold_Switch/2
  Subtract1/1 -> Delay1/1
  Constant/1 -> Threshold_Switch1/3, Threshold_Switch1/1
  Signal_w/1 -> Subtract1/1, Relational Operator2/1, Relational Operator5/1, Abs/1, Add1/1, Relational Operator3/1, Relational Operator7/1
  Relational Operator7/1 -> Threshold_Switch2/2
  Relational Operator1/1 -> Delay5/1
  Threshold_Switch1/1 -> Threshold_Switch2/1
  Threshold_Switch2/1 -> Divide/1
  Length/1 -> Divide/2
  Divide/1 -> Delay7/1
  Delay7/1 -> New_Threshold/1

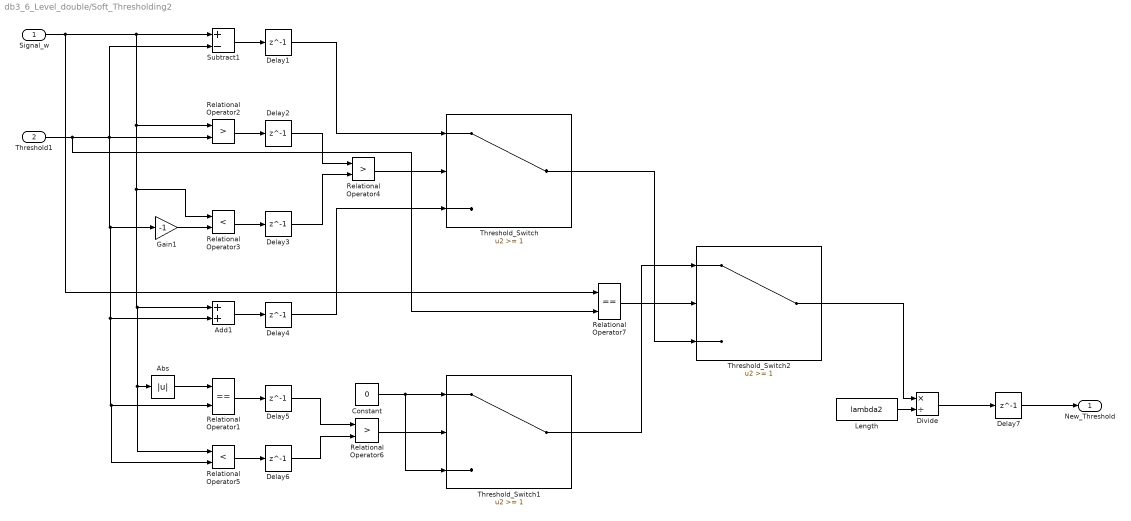
== system db3_6_Level_double/Soft_Thresholding2 ==
  Signal_w : Inport  OutDataTypeStr=double  SampleTime=1/44100
  Threshold1 : Inport  Port=2  OutDataTypeStr=double  SampleTime=1/44100
  Abs : Abs  OutDataTypeStr=double
  Add1 : Sum  AccumDataTypeStr=double  OutDataTypeStr=double
  Constant : Constant  Value=0  OutDataTypeStr=double  SampleTime=1/44100
  Delay{1..7} (7 alike) : Delay  DelayLength=1  SampleTime=1/44100
  Divide : Product  Inputs=*/  OutDataTypeStr=double
  Gain1 : Gain  Gain=-1  ParamDataTypeStr=double  OutMin=-1  OutMax=-0.99  OutDataTypeStr=double
  Length : Constant  Value=lambda2  OutDataTypeStr=double  SampleTime=1/44100
  Relational Operator1 : RelationalOperator  Operator===  OutDataTypeStr=boolean  RndMeth=Simplest
  Relational Operator2 : RelationalOperator  Operator=>  OutDataTypeStr=boolean  RndMeth=Simplest
  Relational Operator3 : RelationalOperator  Operator=<  OutDataTypeStr=boolean  RndMeth=Simplest
  Relational Operator4 : RelationalOperator  Operator=>  OutDataTypeStr=boolean  RndMeth=Simplest
  Relational Operator5 : RelationalOperator  Operator=<  OutDataTypeStr=boolean  RndMeth=Simplest
  Relational Operator6 : RelationalOperator  Operator=>  OutDataTypeStr=boolean  RndMeth=Simplest
  Relational Operator7 : RelationalOperator  Operator===  OutDataTypeStr=boolean  RndMeth=Simplest
  Subtract1 : Sum  Inputs=+-  AccumDataTypeStr=double  OutDataTypeStr=double
  Threshold_Switch : Switch  Threshold=1  OutDataTypeStr=double
  Threshold_Switch1 : Switch  Threshold=1  OutDataTypeStr=double
  Threshold_Switch2 : Switch  Threshold=1  OutDataTypeStr=double
  New_Threshold : Outport  OutDataTypeStr=double  SampleTime=1/44100
  wires:
  Threshold_Switch/1 -> Threshold_Switch2/3
  Relational Operator6/1 -> Threshold_Switch1/2
  Gain1/1 -> Relational Operator3/2
  Delay4/1 -> Threshold_Switch/3
  Add1/1 -> Delay4/1
  Delay2/1 -> Relational Operator4/1
  Delay3/1 -> Relational Operator4/2
  Delay1/1 -> Threshold_Switch/1
  Relational Operator2/1 -> Delay2/1
  Relational Operator3/1 -> Delay3/1
  Relational Operator5/1 -> Delay6/1
  Delay6/1 -> Relational Operator6/2
  Delay5/1 -> Relational Operator6/1
  Threshold1/1 -> Relational Operator2/2, Subtract1/2, Relational Operator5/2, Relational Operator1/2, Add1/2, Gain1/1, Relational Operator7/2
  Abs/1 -> Relational Operator1/1
  Relational Operator4/1 -> Threshold_Switch/2
  Subtract1/1 -> Delay1/1
  Constant/1 -> Threshold_Switch1/3, Threshold_Switch1/1
  Signal_w/1 -> Subtract1/1, Relational Operator2/1, Relational Operator5/1, Abs/1, Add1/1, Relational Operator3/1, Relational Operator7/1
  Relational Operator7/1 -> Threshold_Switch2/2
  Relational Operator1/1 -> Delay5/1
  Threshold_Switch1/1 -> Threshold_Switch2/1
  Threshold_Switch2/1 -> Divide/1
  Length/1 -> Divide/2
  Divide/1 -> Delay7/1
  Delay7/1 -> New_Threshold/1

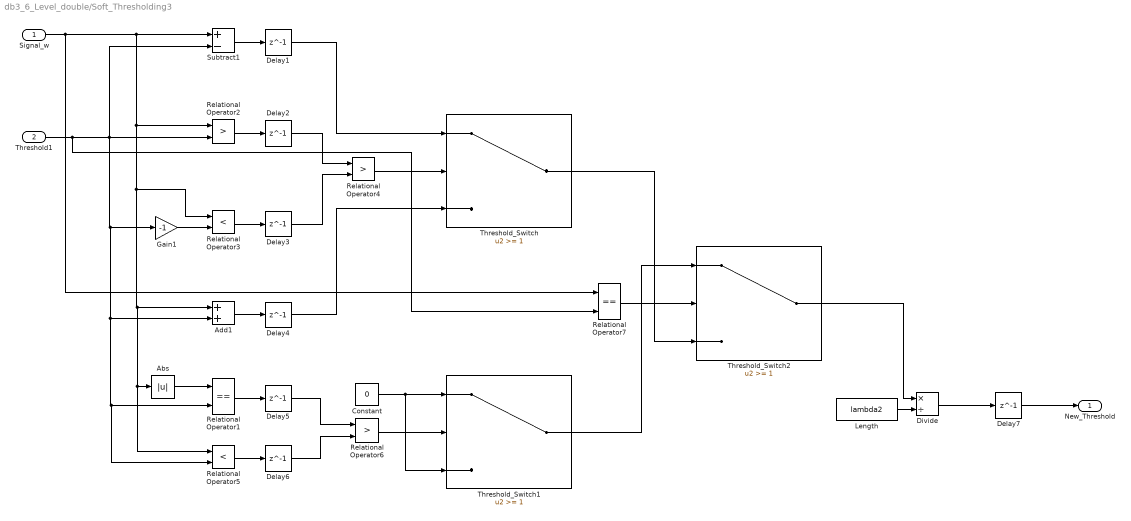
== system db3_6_Level_double/Soft_Thresholding3 ==
  Signal_w : Inport  OutDataTypeStr=double  SampleTime=1/44100
  Threshold1 : Inport  Port=2  OutDataTypeStr=double  SampleTime=1/44100
  Abs : Abs  OutDataTypeStr=double
  Add1 : Sum  AccumDataTypeStr=double  OutDataTypeStr=double
  Constant : Constant  Value=0  OutDataTypeStr=double  SampleTime=1/44100
  Delay{1..7} (7 alike) : Delay  DelayLength=1  SampleTime=1/44100
  Divide : Product  Inputs=*/  OutDataTypeStr=double
  Gain1 : Gain  Gain=-1  ParamDataTypeStr=double  OutMin=-1  OutMax=-0.99  OutDataTypeStr=double
  Length : Constant  Value=lambda2  OutDataTypeStr=double  SampleTime=1/44100
  Relational Operator1 : RelationalOperator  Operator===  OutDataTypeStr=boolean  RndMeth=Simplest
  Relational Operator2 : RelationalOperator  Operator=>  OutDataTypeStr=boolean  RndMeth=Simplest
  Relational Operator3 : RelationalOperator  Operator=<  OutDataTypeStr=boolean  RndMeth=Simplest
  Relational Operator4 : RelationalOperator  Operator=>  OutDataTypeStr=boolean  RndMeth=Simplest
  Relational Operator5 : RelationalOperator  Operator=<  OutDataTypeStr=boolean  RndMeth=Simplest
  Relational Operator6 : RelationalOperator  Operator=>  OutDataTypeStr=boolean  RndMeth=Simplest
  Relational Operator7 : RelationalOperator  Operator===  OutDataTypeStr=boolean  RndMeth=Simplest
  Subtract1 : Sum  Inputs=+-  AccumDataTypeStr=double  OutDataTypeStr=double
  Threshold_Switch : Switch  Threshold=1  OutDataTypeStr=double
  Threshold_Switch1 : Switch  Threshold=1  OutDataTypeStr=double
  Threshold_Switch2 : Switch  Threshold=1  OutDataTypeStr=double
  New_Threshold : Outport  OutDataTypeStr=double  SampleTime=1/44100
  wires:
  Threshold_Switch/1 -> Threshold_Switch2/3
  Relational Operator6/1 -> Threshold_Switch1/2
  Gain1/1 -> Relational Operator3/2
  Delay4/1 -> Threshold_Switch/3
  Add1/1 -> Delay4/1
  Delay2/1 -> Relational Operator4/1
  Delay3/1 -> Relational Operator4/2
  Delay1/1 -> Threshold_Switch/1
  Relational Operator2/1 -> Delay2/1
  Relational Operator3/1 -> Delay3/1
  Relational Operator5/1 -> Delay6/1
  Delay6/1 -> Relational Operator6/2
  Delay5/1 -> Relational Operator6/1
  Threshold1/1 -> Relational Operator2/2, Subtract1/2, Relational Operator5/2, Relational Operator1/2, Add1/2, Gain1/1, Relational Operator7/2
  Abs/1 -> Relational Operator1/1
  Relational Operator4/1 -> Threshold_Switch/2
  Subtract1/1 -> Delay1/1
  Constant/1 -> Threshold_Switch1/3, Threshold_Switch1/1
  Signal_w/1 -> Subtract1/1, Relational Operator2/1, Relational Operator5/1, Abs/1, Add1/1, Relational Operator3/1, Relational Operator7/1
  Relational Operator7/1 -> Threshold_Switch2/2
  Relational Operator1/1 -> Delay5/1
  Threshold_Switch1/1 -> Threshold_Switch2/1
  Threshold_Switch2/1 -> Divide/1
  Length/1 -> Divide/2
  Divide/1 -> Delay7/1
  Delay7/1 -> New_Threshold/1

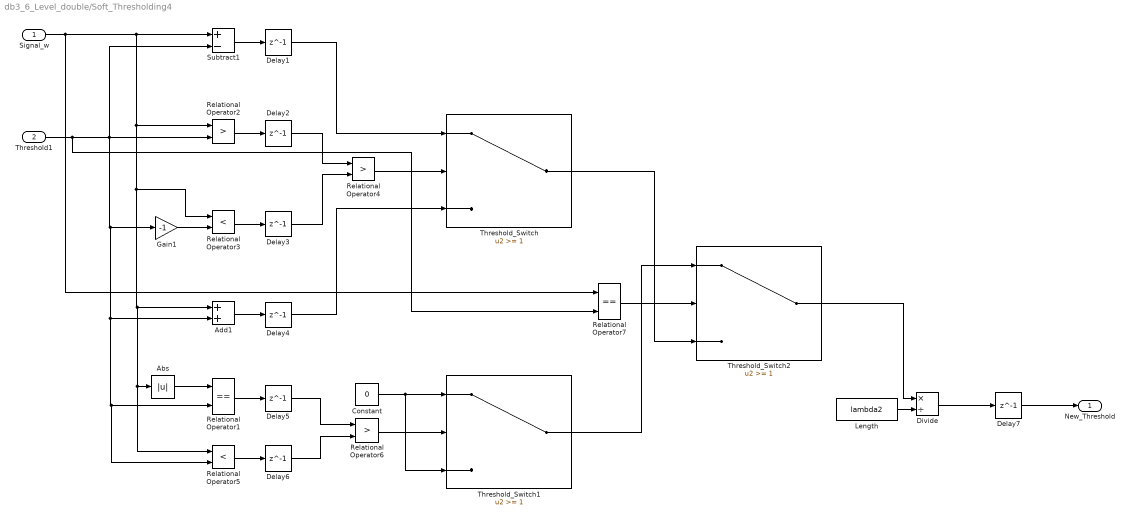
== system db3_6_Level_double/Soft_Thresholding4 ==
  Signal_w : Inport  OutDataTypeStr=double  SampleTime=1/44100
  Threshold1 : Inport  Port=2  OutDataTypeStr=double  SampleTime=1/44100
  Abs : Abs  OutDataTypeStr=double
  Add1 : Sum  AccumDataTypeStr=double  OutDataTypeStr=double
  Constant : Constant  Value=0  OutDataTypeStr=double  SampleTime=1/44100
  Delay{1..7} (7 alike) : Delay  DelayLength=1  SampleTime=1/44100
  Divide : Product  Inputs=*/  OutDataTypeStr=double
  Gain1 : Gain  Gain=-1  ParamDataTypeStr=double  OutMin=-1  OutMax=-0.99  OutDataTypeStr=double
  Length : Constant  Value=lambda2  OutDataTypeStr=double  SampleTime=1/44100
  Relational Operator1 : RelationalOperator  Operator===  OutDataTypeStr=boolean  RndMeth=Simplest
  Relational Operator2 : RelationalOperator  Operator=>  OutDataTypeStr=boolean  RndMeth=Simplest
  Relational Operator3 : RelationalOperator  Operator=<  OutDataTypeStr=boolean  RndMeth=Simplest
  Relational Operator4 : RelationalOperator  Operator=>  OutDataTypeStr=boolean  RndMeth=Simplest
  Relational Operator5 : RelationalOperator  Operator=<  OutDataTypeStr=boolean  RndMeth=Simplest
  Relational Operator6 : RelationalOperator  Operator=>  OutDataTypeStr=boolean  RndMeth=Simplest
  Relational Operator7 : RelationalOperator  Operator===  OutDataTypeStr=boolean  RndMeth=Simplest
  Subtract1 : Sum  Inputs=+-  AccumDataTypeStr=double  OutDataTypeStr=double
  Threshold_Switch : Switch  Threshold=1  OutDataTypeStr=double
  Threshold_Switch1 : Switch  Threshold=1  OutDataTypeStr=double
  Threshold_Switch2 : Switch  Threshold=1  OutDataTypeStr=double
  New_Threshold : Outport  OutDataTypeStr=double  SampleTime=1/44100
  wires:
  Threshold_Switch/1 -> Threshold_Switch2/3
  Relational Operator6/1 -> Threshold_Switch1/2
  Gain1/1 -> Relational Operator3/2
  Delay4/1 -> Threshold_Switch/3
  Add1/1 -> Delay4/1
  Delay2/1 -> Relational Operator4/1
  Delay3/1 -> Relational Operator4/2
  Delay1/1 -> Threshold_Switch/1
  Relational Operator2/1 -> Delay2/1
  Relational Operator3/1 -> Delay3/1
  Relational Operator5/1 -> Delay6/1
  Delay6/1 -> Relational Operator6/2
  Delay5/1 -> Relational Operator6/1
  Threshold1/1 -> Relational Operator2/2, Subtract1/2, Relational Operator5/2, Relational Operator1/2, Add1/2, Gain1/1, Relational Operator7/2
  Abs/1 -> Relational Operator1/1
  Relational Operator4/1 -> Threshold_Switch/2
  Subtract1/1 -> Delay1/1
  Constant/1 -> Threshold_Switch1/3, Threshold_Switch1/1
  Signal_w/1 -> Subtract1/1, Relational Operator2/1, Relational Operator5/1, Abs/1, Add1/1, Relational Operator3/1, Relational Operator7/1
  Relational Operator7/1 -> Threshold_Switch2/2
  Relational Operator1/1 -> Delay5/1
  Threshold_Switch1/1 -> Threshold_Switch2/1
  Threshold_Switch2/1 -> Divide/1
  Length/1 -> Divide/2
  Divide/1 -> Delay7/1
  Delay7/1 -> New_Threshold/1

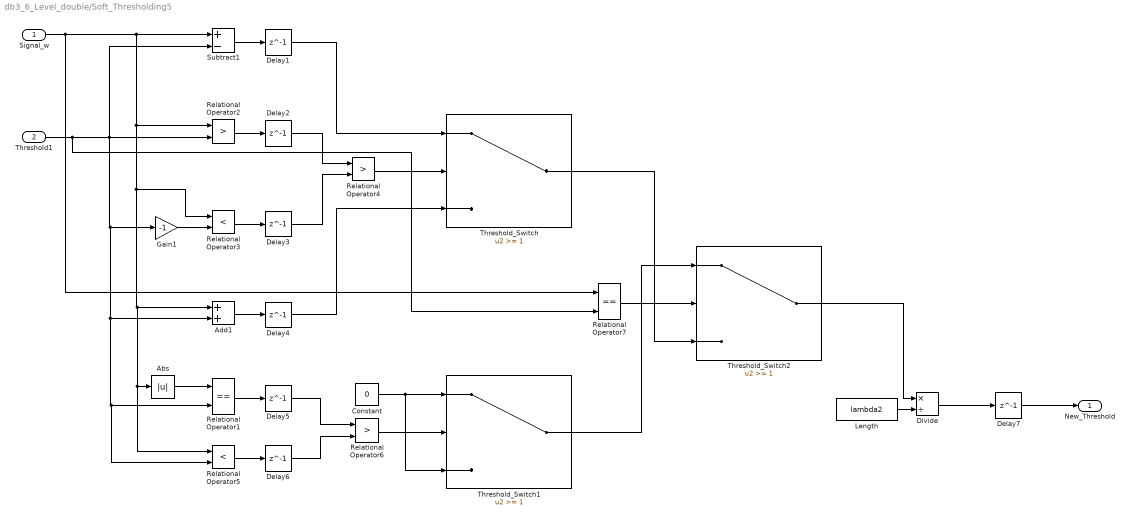
== system db3_6_Level_double/Soft_Thresholding5 ==
  Signal_w : Inport  OutDataTypeStr=double  SampleTime=1/44100
  Threshold1 : Inport  Port=2  OutDataTypeStr=double  SampleTime=1/44100
  Abs : Abs  OutDataTypeStr=double
  Add1 : Sum  AccumDataTypeStr=double  OutDataTypeStr=double
  Constant : Constant  Value=0  OutDataTypeStr=double  SampleTime=1/44100
  Delay{1..7} (7 alike) : Delay  DelayLength=1  SampleTime=1/44100
  Divide : Product  Inputs=*/  OutDataTypeStr=double
  Gain1 : Gain  Gain=-1  ParamDataTypeStr=double  OutMin=-1  OutMax=-0.99  OutDataTypeStr=double
  Length : Constant  Value=lambda2  OutDataTypeStr=double  SampleTime=1/44100
  Relational Operator1 : RelationalOperator  Operator===  OutDataTypeStr=boolean  RndMeth=Simplest
  Relational Operator2 : RelationalOperator  Operator=>  OutDataTypeStr=boolean  RndMeth=Simplest
  Relational Operator3 : RelationalOperator  Operator=<  OutDataTypeStr=boolean  RndMeth=Simplest
  Relational Operator4 : RelationalOperator  Operator=>  OutDataTypeStr=boolean  RndMeth=Simplest
  Relational Operator5 : RelationalOperator  Operator=<  OutDataTypeStr=boolean  RndMeth=Simplest
  Relational Operator6 : RelationalOperator  Operator=>  OutDataTypeStr=boolean  RndMeth=Simplest
  Relational Operator7 : RelationalOperator  Operator===  OutDataTypeStr=boolean  RndMeth=Simplest
  Subtract1 : Sum  Inputs=+-  AccumDataTypeStr=double  OutDataTypeStr=double
  Threshold_Switch : Switch  Threshold=1  OutDataTypeStr=double
  Threshold_Switch1 : Switch  Threshold=1  OutDataTypeStr=double
  Threshold_Switch2 : Switch  Threshold=1  OutDataTypeStr=double
  New_Threshold : Outport  OutDataTypeStr=double  SampleTime=1/44100
  wires:
  Threshold_Switch/1 -> Threshold_Switch2/3
  Relational Operator6/1 -> Threshold_Switch1/2
  Gain1/1 -> Relational Operator3/2
  Delay4/1 -> Threshold_Switch/3
  Add1/1 -> Delay4/1
  Delay2/1 -> Relational Operator4/1
  Delay3/1 -> Relational Operator4/2
  Delay1/1 -> Threshold_Switch/1
  Relational Operator2/1 -> Delay2/1
  Relational Operator3/1 -> Delay3/1
  Relational Operator5/1 -> Delay6/1
  Delay6/1 -> Relational Operator6/2
  Delay5/1 -> Relational Operator6/1
  Threshold1/1 -> Relational Operator2/2, Subtract1/2, Relational Operator5/2, Relational Operator1/2, Add1/2, Gain1/1, Relational Operator7/2
  Abs/1 -> Relational Operator1/1
  Relational Operator4/1 -> Threshold_Switch/2
  Subtract1/1 -> Delay1/1
  Constant/1 -> Threshold_Switch1/3, Threshold_Switch1/1
  Signal_w/1 -> Subtract1/1, Relational Operator2/1, Relational Operator5/1, Abs/1, Add1/1, Relational Operator3/1, Relational Operator7/1
  Relational Operator7/1 -> Threshold_Switch2/2
  Relational Operator1/1 -> Delay5/1
  Threshold_Switch1/1 -> Threshold_Switch2/1
  Threshold_Switch2/1 -> Divide/1
  Length/1 -> Divide/2
  Divide/1 -> Delay7/1
  Delay7/1 -> New_Threshold/1

== system db3_6_Level_double/Threshold_Estimator ==
  Signal_w : Inport  OutDataTypeStr=double  SampleTime=1/44100
  Absolute_Value1 : Subsystem
  Length : Constant  Value=lambda2  OutDataTypeStr=double  SampleTime=1/44100
  Median2 : Subsystem
  Multiply : Product  OutDataTypeStr=double
  Threshold : Outport  OutDataTypeStr=double  SampleTime=1/44100  VectorParamsAs1DForOutWhenUnconnected=off
  wires:
  Length/1 -> Multiply/2
  Median2/1(Median) -> Multiply/1
  Absolute_Value1/1(Out_Abs) -> Median2/1(Signal_w3)
  Signal_w/1 -> Absolute_Value1/1(Signal_w4)
  Multiply/1 -> Threshold/1

== system db3_6_Level_double/1st_Level_Decomp/HiD_Even ==
  In_HiD_e : Inport  OutDataTypeStr=double  SampleTime=1/44100
  Add : Sum  AccumDataTypeStr=double  OutDataTypeStr=double
  Add1 : Sum  AccumDataTypeStr=double  OutDataTypeStr=double
  Delay{,1..3} (4 alike) : Delay  DelayLength=1  SampleTime=1/44100
  HiD_0 : Constant  Value=-0.332670553  OutDataTypeStr=double  SampleTime=1/44100
  HiD_2 : Constant  Value=-0.459877502  OutDataTypeStr=double  SampleTime=1/44100
  HiD_4 : Constant  Value=0.085441274  OutDataTypeStr=double  SampleTime=1/44100
  Multiply : Product  OutDataTypeStr=double
  Multiply1 : Product  OutDataTypeStr=double
  Multiply2 : Product  OutDataTypeStr=double
  Rate Transition : RateTransition  OutPortSampleTime=1/44100
  Rate Transition1 : RateTransition  OutPortSampleTime=1/44100
  Out_HiD_e : Outport  OutDataTypeStr=double  SampleTime=1/44100  VectorParamsAs1DForOutWhenUnconnected=off
  wires:
  In_HiD_e/1 -> Delay/1, Multiply/2
  Rate Transition/1 -> Delay1/1, Multiply1/2
  HiD_0/1 -> Multiply/1
  HiD_2/1 -> Multiply1/1
  Add/1 -> Out_HiD_e/1
  Rate Transition1/1 -> Multiply2/2
  HiD_4/1 -> Multiply2/1
  Multiply1/1 -> Add1/1
  Multiply2/1 -> Delay2/1
  Delay2/1 -> Add1/2
  Add1/1 -> Delay3/1
  Delay3/1 -> Add/2
  Multiply/1 -> Add/1
  Delay/1 -> Rate Transition/1
  Delay1/1 -> Rate Transition1/1

== system db3_6_Level_double/1st_Level_Decomp/HiD_Odd ==
  In_HiD_o : Inport  OutDataTypeStr=double  SampleTime=1/44100
  Add : Sum  AccumDataTypeStr=double  OutDataTypeStr=double
  Add1 : Sum  AccumDataTypeStr=double  OutDataTypeStr=double
  Delay{,1..3} (4 alike) : Delay  DelayLength=1  SampleTime=1/44100
  HiD_1 : Constant  Value=0.806891509  OutDataTypeStr=double  SampleTime=1/44100
  HiD_3 : Constant  Value=-0.13501102  OutDataTypeStr=double  SampleTime=1/44100
  HiD_5 : Constant  Value=0.035226292  OutDataTypeStr=double  SampleTime=1/44100
  Multiply : Product  OutDataTypeStr=double
  Multiply1 : Product  OutDataTypeStr=double
  Multiply2 : Product  OutDataTypeStr=double
  Rate Transition : RateTransition  OutPortSampleTime=1/44100
  Rate Transition1 : RateTransition  OutPortSampleTime=1/44100
  Out_HiD_o : Outport  OutDataTypeStr=double  SampleTime=1/44100  VectorParamsAs1DForOutWhenUnconnected=off
  wires:
  HiD_5/1 -> Multiply2/1
  HiD_3/1 -> Multiply1/1
  Add/1 -> Out_HiD_o/1
  Delay2/1 -> Add1/2
  Delay3/1 -> Add/2
  Add1/1 -> Delay3/1
  Multiply/1 -> Add/1
  HiD_1/1 -> Multiply/1
  Rate Transition/1 -> Delay1/1, Multiply1/2
  Multiply1/1 -> Add1/1
  Multiply2/1 -> Delay2/1
  Rate Transition1/1 -> Multiply2/2
  In_HiD_o/1 -> Multiply/2, Delay/1
  Delay/1 -> Rate Transition/1
  Delay1/1 -> Rate Transition1/1

== system db3_6_Level_double/1st_Level_Decomp/LoD_Even ==
  In_LoD_e : Inport  OutDataTypeStr=double  SampleTime=1/44100
  Add : Sum  AccumDataTypeStr=double  OutDataTypeStr=double
  Add1 : Sum  AccumDataTypeStr=double  OutDataTypeStr=double
  Delay{,1..3} (4 alike) : Delay  DelayLength=1  SampleTime=1/44100
  LoD_0 : Constant  Value=0.035226292  OutDataTypeStr=double  SampleTime=1/44100
  LoD_2 : Constant  Value=-0.13501102  OutDataTypeStr=double  SampleTime=1/44100
  LoD_4 : Constant  Value=0.806891509  OutDataTypeStr=double  SampleTime=1/44100
  Multiply : Product  OutDataTypeStr=double
  Multiply1 : Product  OutDataTypeStr=double
  Multiply2 : Product  OutDataTypeStr=double
  Rate Transition : RateTransition  OutPortSampleTime=1/44100
  Rate Transition1 : RateTransition  OutPortSampleTime=1/44100
  Out_LoD_e : Outport  OutDataTypeStr=double  SampleTime=1/44100  VectorParamsAs1DForOutWhenUnconnected=off
  wires:
  LoD_4/1 -> Multiply2/1
  LoD_2/1 -> Multiply1/1
  Add/1 -> Out_LoD_e/1
  Delay2/1 -> Add1/2
  Delay3/1 -> Add/2
  Add1/1 -> Delay3/1
  Multiply/1 -> Add/1
  LoD_0/1 -> Multiply/1
  Rate Transition/1 -> Delay1/1, Multiply1/2
  Multiply1/1 -> Add1/1
  Multiply2/1 -> Delay2/1
  Rate Transition1/1 -> Multiply2/2
  In_LoD_e/1 -> Delay/1, Multiply/2
  Delay/1 -> Rate Transition/1
  Delay1/1 -> Rate Transition1/1

== system db3_6_Level_double/1st_Level_Decomp/LoD_Odd ==
  In_LoD_o : Inport  OutDataTypeStr=double  SampleTime=1/44100
  Add : Sum  AccumDataTypeStr=double  OutDataTypeStr=double
  Add1 : Sum  AccumDataTypeStr=double  OutDataTypeStr=double
  Delay{,1..3} (4 alike) : Delay  DelayLength=1  SampleTime=1/44100
  LoD_1 : Constant  Value=-0.085441274  OutDataTypeStr=double  SampleTime=1/44100
  LoD_3 : Constant  Value=0.459877502  OutDataTypeStr=double  SampleTime=1/44100
  LoD_5 : Constant  Value=0.332670553  OutDataTypeStr=double  SampleTime=1/44100
  Multiply : Product  OutDataTypeStr=double
  Multiply1 : Product  OutDataTypeStr=double
  Multiply2 : Product  OutDataTypeStr=double
  Rate Transition : RateTransition  OutPortSampleTime=1/44100
  Rate Transition1 : RateTransition  OutPortSampleTime=1/44100
  Out_LoD_o : Outport  OutDataTypeStr=double  SampleTime=1/44100  VectorParamsAs1DForOutWhenUnconnected=off
  wires:
  LoD_5/1 -> Multiply2/1
  LoD_3/1 -> Multiply1/1
  Add/1 -> Out_LoD_o/1
  Delay2/1 -> Add1/2
  Delay3/1 -> Add/2
  Add1/1 -> Delay3/1
  Multiply/1 -> Add/1
  LoD_1/1 -> Multiply/1
  Rate Transition/1 -> Delay1/1, Multiply1/2
  Multiply1/1 -> Add1/1
  Multiply2/1 -> Delay2/1
  Rate Transition1/1 -> Multiply2/2
  In_LoD_o/1 -> Delay/1, Multiply/2
  Delay/1 -> Rate Transition/1
  Delay1/1 -> Rate Transition1/1

== system db3_6_Level_double/1st_Level_Recon/HiR_Even ==
  In_HiR_e : Inport  OutDataTypeStr=double  SampleTime=1/44100
  Add : Sum  AccumDataTypeStr=double  OutDataTypeStr=double
  Add1 : Sum  AccumDataTypeStr=double  OutDataTypeStr=double
  Delay : Delay  DelayLength=1  SampleTime=1/44100
  Delay1 : Delay  DelayLength=1  SampleTime=1/44100
  Delay2 : Delay  DelayLength=1  SampleTime=0.000022675736
  Delay3 : Delay  DelayLength=1  SampleTime=0.000022675736
  HiR_0 : Constant  Value=0.035226292  OutDataTypeStr=double  SampleTime=1/44100
  HiR_2 : Constant  Value=-0.13501102  OutDataTypeStr=double  SampleTime=1/44100
  HiR_4 : Constant  Value=0.806891509  OutDataTypeStr=double  SampleTime=1/44100
  Multiply : Product  OutDataTypeStr=double
  Multiply1 : Product  OutDataTypeStr=double
  Multiply2 : Product  OutDataTypeStr=double
  Rate Transition : RateTransition  OutPortSampleTime=1/44100
  Rate Transition1 : RateTransition  OutPortSampleTime=1/44100
  Out_HiR_e : Outport  OutDataTypeStr=double  SampleTime=1/44100  VectorParamsAs1DForOutWhenUnconnected=off
  wires:
  Delay3/1 -> Add/2
  In_HiR_e/1 -> Delay/1, Multiply/2
  HiR_4/1 -> Multiply2/1
  Multiply/1 -> Add/1
  Add1/1 -> Delay3/1
  Multiply2/1 -> Delay2/1
  Multiply1/1 -> Add1/1
  Delay2/1 -> Add1/2
  Add/1 -> Out_HiR_e/1
  HiR_0/1 -> Multiply/1
  HiR_2/1 -> Multiply1/1
  Delay1/1 -> Rate Transition1/1
  Rate Transition/1 -> Delay1/1, Multiply1/2
  Rate Transition1/1 -> Multiply2/2
  Delay/1 -> Rate Transition/1
